simulink model "fsfc_bias_est"  (R2023b)
settings: Solver=FixedStepAuto  StartTime=0.0  StopTime=SIMTIME  FixedStep=SIMSTEP  RelTol=1e-3
values from neighbouring files (symbols this model uses):
  A = [z33,    eye(3) ... (first row only)    [smol_boat.m]
  Aa = [A, Bv; zeros(3, 6), z33]    [smol_boat.m]
  B = [z33, inv(M)]'    [smol_boat.m]
  Ba = [B;z33]    [smol_boat.m]
  bias = [bias_X;0;0]    [smol_boat.m]
  Bv = [z33, inv(M)]'    [smol_boat.m]
  C = [eye(n_outputs,n_states)]    [smol_boat.m]
  Ca = [C, z33]    [smol_boat.m]
  K1 = Kt1*Q    [smol_boat.m]
  L = 90    [loadvars_smol_boat.m]    (also in smol_boat.m = place(Aa', Ca', lambda_obs)')
  ref = zeros(n_outputs, 1)    [smol_boat.m]
  x0 = zeros(n_states,1)    [smol_boat.m]
  xhat_0 = zeros(n_states+n_aug,1)    [smol_boat.m]
settings Model: Creator=Lorenzo-Desk  LastModifiedBy=Lorenzo-Desk
settings DataIOCC: ReturnWorkspaceOutputs=off

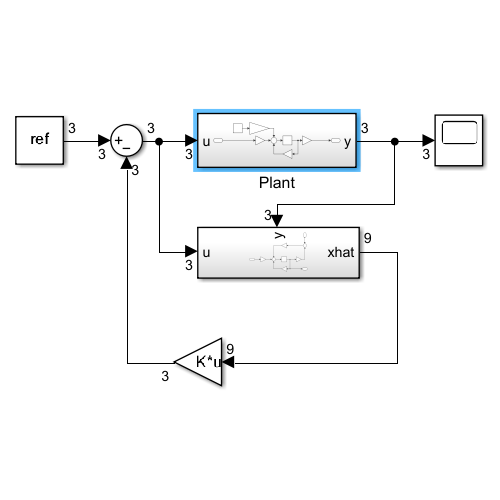
[thumbnail: Simulink's stored preview of the top-level diagram]
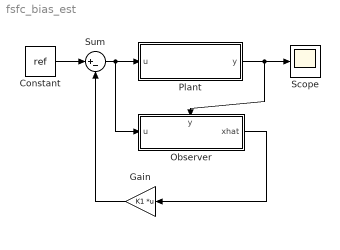
== system fsfc_bias_est ==
  Constant : Constant  Value=ref
  Gain : Gain  Gain=K1  Multiplication=Matrix(K*u)
  Observer : Subsystem
      settings: PortSchema="{\"entries\":[{\"content\":{\"sides\":[{\"content\":{\"connectorIds\":[\"In1\"]},\"type\":\"ConnectorPlacement.EquallySpacedRectSide\",\"uuid\":\"73eb13a4-821c-44f7-a0c5-8658f41102da\"},{\"content\":{\"connectorIds\":[\"Out1\"],\"side\":\"RIGHT\"},\"type\":\"ConnectorPlacement.EquallySpacedRectSide\",\"uuid\":\"46a10ada-d417-4d5f-8fe2-bf3b9a741608\"},{\"content\":{\"connectorIds\":[\"In2\"],\"side\":\"TOP\"},\"type\":\"ConnectorPlacement.EquallySpacedRectSide\",\"uuid\":\"761d0b5b-7137-4372-8030-4ca1ce843623\"}]},\"type\":\"ConnectorPlacement.EquallySpacedConnector\",\"uuid\":\"cfec28aa-9991-4d83-9aa1-5597ff8e72d9\"}],\"packageUris\":[\"http://schema.mathworks.com/mf0/Connector/R2020b\"],\"version\":\"1.0\"}"
  Plant : Subsystem
  Scope : Scope
  Sum : Sum  Inputs=|+-
  wires:
  Plant/1(y) -> Scope/1, Observer/2(y)
  Sum/1 -> Observer/1(u), Plant/1(u)
  Observer/1(xhat) -> Gain/1
  Constant/1 -> Sum/1
  Gain/1 -> Sum/2

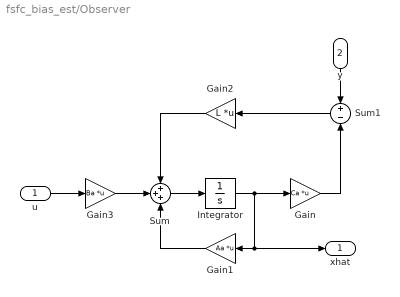
== system fsfc_bias_est/Observer ==
  u : Inport
  y : Inport  Port=2
  Gain : Gain  Gain=Ca  Multiplication=Matrix(K*u)
  Gain1 : Gain  Gain=Aa  Multiplication=Matrix(K*u)
  Gain2 : Gain  Gain=L  Multiplication=Matrix(K*u)
  Gain3 : Gain  Gain=Ba  Multiplication=Matrix(K*u)
  Integrator : Integrator  InitialCondition=xhat_0
  Sum : Sum  Inputs=+++
  Sum1 : Sum  Inputs=+|-
  xhat : Outport
  wires:
  Integrator/1 -> xhat/1, Gain1/1, Gain/1
  Sum/1 -> Integrator/1
  Gain2/1 -> Sum/1
  Gain/1 -> Sum1/2
  Sum1/1 -> Gain2/1
  Gain1/1 -> Sum/3
  Gain3/1 -> Sum/2
  u/1 -> Gain3/1
  y/1 -> Sum1/1

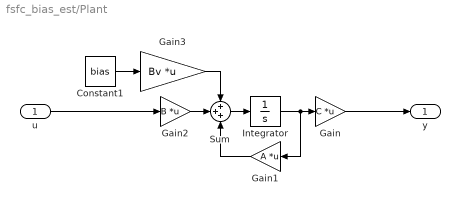
== system fsfc_bias_est/Plant ==
  u : Inport
  Constant1 : Constant  Value=bias
  Gain : Gain  Gain=C  Multiplication=Matrix(K*u) (u vector)
  Gain1 : Gain  Gain=A  Multiplication=Matrix(K*u) (u vector)
  Gain2 : Gain  Gain=B  Multiplication=Matrix(K*u) (u vector)
  Gain3 : Gain  Gain=Bv  Multiplication=Matrix(K*u) (u vector)
  Integrator : Integrator  InitialCondition=x0
  Sum : Sum  Inputs=+++
  y : Outport
  wires:
  Gain3/1 -> Sum/1
  Integrator/1 -> Gain/1, Gain1/1
  Gain2/1 -> Sum/2
  Constant1/1 -> Gain3/1
  Sum/1 -> Integrator/1
  Gain/1 -> y/1
  Gain1/1 -> Sum/3
  u/1 -> Gain2/1
